simulink library "lib_rfsoc_fec"  (R2020b)
settings: Solver=VariableStepAuto  StartTime=0.0  StopTime=10.0  RelTol=1e-3
undefined symbols (not defined in the file): d, fs, generator_polynomial
libraries: hdlsllib x114, commseqgen3 x84, simulink x22, dspsigops x13, $bdroot x2
(part 4 of 5)

== system lib_rfsoc_fec/QAM Mapping/QAM Mapping/N-Width QAM-16 Symbol Mapping Imag/QAM-16 Symbol Mapping 11 ==
  bits : Inport
  Bit Slice1 : hdlsllib/Logic and Bit Operations/Bit Slice  lidx=n+1  ridx=n
      settings: SourceProductBaseCode=SL
  Constant1 : Constant  Value=3  OutDataTypeStr=fixdt(1,3,0)  SampleTime=-1
  Constant2 : Constant  OutDataTypeStr=fixdt(1,3,0)  SampleTime=-1
  Constant3 : Constant  Value=-1  OutDataTypeStr=fixdt(1,3,0)  SampleTime=-1
  Constant4 : Constant  Value=-3  OutDataTypeStr=fixdt(1,3,0)  SampleTime=-1
  Multiport Switch1 : MultiPortSwitch  DataPortOrder=Zero-based contiguous  Inputs=4  zeroidx=on
  Q : Outport
  wires:
  Bit Slice1/1 -> Multiport Switch1/1
  Multiport Switch1/1 -> Q/1
  bits/1 -> Bit Slice1/1
  Constant3/1 -> Multiport Switch1/5
  Constant4/1 -> Multiport Switch1/4
  Constant1/1 -> Multiport Switch1/2
  Constant2/1 -> Multiport Switch1/3

== system lib_rfsoc_fec/QAM Mapping/QAM Mapping/N-Width QAM-16 Symbol Mapping Imag/QAM-16 Symbol Mapping 12 ==
  bits : Inport
  Bit Slice1 : hdlsllib/Logic and Bit Operations/Bit Slice  lidx=n+1  ridx=n
      settings: SourceProductBaseCode=SL
  Constant1 : Constant  Value=3  OutDataTypeStr=fixdt(1,3,0)  SampleTime=-1
  Constant2 : Constant  OutDataTypeStr=fixdt(1,3,0)  SampleTime=-1
  Constant3 : Constant  Value=-1  OutDataTypeStr=fixdt(1,3,0)  SampleTime=-1
  Constant4 : Constant  Value=-3  OutDataTypeStr=fixdt(1,3,0)  SampleTime=-1
  Multiport Switch1 : MultiPortSwitch  DataPortOrder=Zero-based contiguous  Inputs=4  zeroidx=on
  Q : Outport
  wires:
  Bit Slice1/1 -> Multiport Switch1/1
  Multiport Switch1/1 -> Q/1
  bits/1 -> Bit Slice1/1
  Constant3/1 -> Multiport Switch1/5
  Constant4/1 -> Multiport Switch1/4
  Constant1/1 -> Multiport Switch1/2
  Constant2/1 -> Multiport Switch1/3

== system lib_rfsoc_fec/QAM Mapping/QAM Mapping/N-Width QAM-16 Symbol Mapping Imag/QAM-16 Symbol Mapping 13 ==
  bits : Inport
  Bit Slice1 : hdlsllib/Logic and Bit Operations/Bit Slice  lidx=n+1  ridx=n
      settings: SourceProductBaseCode=SL
  Constant1 : Constant  Value=3  OutDataTypeStr=fixdt(1,3,0)  SampleTime=-1
  Constant2 : Constant  OutDataTypeStr=fixdt(1,3,0)  SampleTime=-1
  Constant3 : Constant  Value=-1  OutDataTypeStr=fixdt(1,3,0)  SampleTime=-1
  Constant4 : Constant  Value=-3  OutDataTypeStr=fixdt(1,3,0)  SampleTime=-1
  Multiport Switch1 : MultiPortSwitch  DataPortOrder=Zero-based contiguous  Inputs=4  zeroidx=on
  Q : Outport
  wires:
  Bit Slice1/1 -> Multiport Switch1/1
  Multiport Switch1/1 -> Q/1
  bits/1 -> Bit Slice1/1
  Constant3/1 -> Multiport Switch1/5
  Constant4/1 -> Multiport Switch1/4
  Constant1/1 -> Multiport Switch1/2
  Constant2/1 -> Multiport Switch1/3

== system lib_rfsoc_fec/QAM Mapping/QAM Mapping/N-Width QAM-16 Symbol Mapping Imag/QAM-16 Symbol Mapping 14 ==
  bits : Inport
  Bit Slice1 : hdlsllib/Logic and Bit Operations/Bit Slice  lidx=n+1  ridx=n
      settings: SourceProductBaseCode=SL
  Constant1 : Constant  Value=3  OutDataTypeStr=fixdt(1,3,0)  SampleTime=-1
  Constant2 : Constant  OutDataTypeStr=fixdt(1,3,0)  SampleTime=-1
  Constant3 : Constant  Value=-1  OutDataTypeStr=fixdt(1,3,0)  SampleTime=-1
  Constant4 : Constant  Value=-3  OutDataTypeStr=fixdt(1,3,0)  SampleTime=-1
  Multiport Switch1 : MultiPortSwitch  DataPortOrder=Zero-based contiguous  Inputs=4  zeroidx=on
  Q : Outport
  wires:
  Bit Slice1/1 -> Multiport Switch1/1
  Multiport Switch1/1 -> Q/1
  bits/1 -> Bit Slice1/1
  Constant3/1 -> Multiport Switch1/5
  Constant4/1 -> Multiport Switch1/4
  Constant1/1 -> Multiport Switch1/2
  Constant2/1 -> Multiport Switch1/3

== system lib_rfsoc_fec/QAM Mapping/QAM Mapping/N-Width QAM-16 Symbol Mapping Imag/QAM-16 Symbol Mapping 15 ==
  bits : Inport
  Bit Slice1 : hdlsllib/Logic and Bit Operations/Bit Slice  lidx=n+1  ridx=n
      settings: SourceProductBaseCode=SL
  Constant1 : Constant  Value=3  OutDataTypeStr=fixdt(1,3,0)  SampleTime=-1
  Constant2 : Constant  OutDataTypeStr=fixdt(1,3,0)  SampleTime=-1
  Constant3 : Constant  Value=-1  OutDataTypeStr=fixdt(1,3,0)  SampleTime=-1
  Constant4 : Constant  Value=-3  OutDataTypeStr=fixdt(1,3,0)  SampleTime=-1
  Multiport Switch1 : MultiPortSwitch  DataPortOrder=Zero-based contiguous  Inputs=4  zeroidx=on
  Q : Outport
  wires:
  Bit Slice1/1 -> Multiport Switch1/1
  Multiport Switch1/1 -> Q/1
  bits/1 -> Bit Slice1/1
  Constant3/1 -> Multiport Switch1/5
  Constant4/1 -> Multiport Switch1/4
  Constant1/1 -> Multiport Switch1/2
  Constant2/1 -> Multiport Switch1/3

== system lib_rfsoc_fec/QAM Mapping/QAM Mapping/N-Width QAM-16 Symbol Mapping Imag/QAM-16 Symbol Mapping 16 ==
  bits : Inport
  Bit Slice1 : hdlsllib/Logic and Bit Operations/Bit Slice  lidx=n+1  ridx=n
      settings: SourceProductBaseCode=SL
  Constant1 : Constant  Value=3  OutDataTypeStr=fixdt(1,3,0)  SampleTime=-1
  Constant2 : Constant  OutDataTypeStr=fixdt(1,3,0)  SampleTime=-1
  Constant3 : Constant  Value=-1  OutDataTypeStr=fixdt(1,3,0)  SampleTime=-1
  Constant4 : Constant  Value=-3  OutDataTypeStr=fixdt(1,3,0)  SampleTime=-1
  Multiport Switch1 : MultiPortSwitch  DataPortOrder=Zero-based contiguous  Inputs=4  zeroidx=on
  Q : Outport
  wires:
  Bit Slice1/1 -> Multiport Switch1/1
  Multiport Switch1/1 -> Q/1
  bits/1 -> Bit Slice1/1
  Constant3/1 -> Multiport Switch1/5
  Constant4/1 -> Multiport Switch1/4
  Constant1/1 -> Multiport Switch1/2
  Constant2/1 -> Multiport Switch1/3

== system lib_rfsoc_fec/QAM Mapping/QAM Mapping/N-Width QAM-16 Symbol Mapping Imag/QAM-16 Symbol Mapping 17 ==
  bits : Inport
  Bit Slice1 : hdlsllib/Logic and Bit Operations/Bit Slice  lidx=n+1  ridx=n
      settings: SourceProductBaseCode=SL
  Constant1 : Constant  Value=3  OutDataTypeStr=fixdt(1,3,0)  SampleTime=-1
  Constant2 : Constant  OutDataTypeStr=fixdt(1,3,0)  SampleTime=-1
  Constant3 : Constant  Value=-1  OutDataTypeStr=fixdt(1,3,0)  SampleTime=-1
  Constant4 : Constant  Value=-3  OutDataTypeStr=fixdt(1,3,0)  SampleTime=-1
  Multiport Switch1 : MultiPortSwitch  DataPortOrder=Zero-based contiguous  Inputs=4  zeroidx=on
  Q : Outport
  wires:
  Bit Slice1/1 -> Multiport Switch1/1
  Multiport Switch1/1 -> Q/1
  bits/1 -> Bit Slice1/1
  Constant3/1 -> Multiport Switch1/5
  Constant4/1 -> Multiport Switch1/4
  Constant1/1 -> Multiport Switch1/2
  Constant2/1 -> Multiport Switch1/3

== system lib_rfsoc_fec/QAM Mapping/QAM Mapping/N-Width QAM-16 Symbol Mapping Imag/QAM-16 Symbol Mapping 18 ==
  bits : Inport
  Bit Slice1 : hdlsllib/Logic and Bit Operations/Bit Slice  lidx=n+1  ridx=n
      settings: SourceProductBaseCode=SL
  Constant1 : Constant  Value=3  OutDataTypeStr=fixdt(1,3,0)  SampleTime=-1
  Constant2 : Constant  OutDataTypeStr=fixdt(1,3,0)  SampleTime=-1
  Constant3 : Constant  Value=-1  OutDataTypeStr=fixdt(1,3,0)  SampleTime=-1
  Constant4 : Constant  Value=-3  OutDataTypeStr=fixdt(1,3,0)  SampleTime=-1
  Multiport Switch1 : MultiPortSwitch  DataPortOrder=Zero-based contiguous  Inputs=4  zeroidx=on
  Q : Outport
  wires:
  Bit Slice1/1 -> Multiport Switch1/1
  Multiport Switch1/1 -> Q/1
  bits/1 -> Bit Slice1/1
  Constant3/1 -> Multiport Switch1/5
  Constant4/1 -> Multiport Switch1/4
  Constant1/1 -> Multiport Switch1/2
  Constant2/1 -> Multiport Switch1/3

== system lib_rfsoc_fec/QAM Mapping/QAM Mapping/N-Width QAM-16 Symbol Mapping Imag/QAM-16 Symbol Mapping 19 ==
  bits : Inport
  Bit Slice1 : hdlsllib/Logic and Bit Operations/Bit Slice  lidx=n+1  ridx=n
      settings: SourceProductBaseCode=SL
  Constant1 : Constant  Value=3  OutDataTypeStr=fixdt(1,3,0)  SampleTime=-1
  Constant2 : Constant  OutDataTypeStr=fixdt(1,3,0)  SampleTime=-1
  Constant3 : Constant  Value=-1  OutDataTypeStr=fixdt(1,3,0)  SampleTime=-1
  Constant4 : Constant  Value=-3  OutDataTypeStr=fixdt(1,3,0)  SampleTime=-1
  Multiport Switch1 : MultiPortSwitch  DataPortOrder=Zero-based contiguous  Inputs=4  zeroidx=on
  Q : Outport
  wires:
  Bit Slice1/1 -> Multiport Switch1/1
  Multiport Switch1/1 -> Q/1
  bits/1 -> Bit Slice1/1
  Constant3/1 -> Multiport Switch1/5
  Constant4/1 -> Multiport Switch1/4
  Constant1/1 -> Multiport Switch1/2
  Constant2/1 -> Multiport Switch1/3

== system lib_rfsoc_fec/QAM Mapping/QAM Mapping/N-Width QAM-16 Symbol Mapping Imag/QAM-16 Symbol Mapping 2 ==
  bits : Inport
  Bit Slice1 : hdlsllib/Logic and Bit Operations/Bit Slice  lidx=n+1  ridx=n
      settings: SourceProductBaseCode=SL
  Constant1 : Constant  Value=3  OutDataTypeStr=fixdt(1,3,0)  SampleTime=-1
  Constant2 : Constant  OutDataTypeStr=fixdt(1,3,0)  SampleTime=-1
  Constant3 : Constant  Value=-1  OutDataTypeStr=fixdt(1,3,0)  SampleTime=-1
  Constant4 : Constant  Value=-3  OutDataTypeStr=fixdt(1,3,0)  SampleTime=-1
  Multiport Switch1 : MultiPortSwitch  DataPortOrder=Zero-based contiguous  Inputs=4  zeroidx=on
  Q : Outport
  wires:
  Bit Slice1/1 -> Multiport Switch1/1
  Multiport Switch1/1 -> Q/1
  bits/1 -> Bit Slice1/1
  Constant3/1 -> Multiport Switch1/5
  Constant4/1 -> Multiport Switch1/4
  Constant1/1 -> Multiport Switch1/2
  Constant2/1 -> Multiport Switch1/3

== system lib_rfsoc_fec/QAM Mapping/QAM Mapping/N-Width QAM-16 Symbol Mapping Imag/QAM-16 Symbol Mapping 20 ==
  bits : Inport
  Bit Slice1 : hdlsllib/Logic and Bit Operations/Bit Slice  lidx=n+1  ridx=n
      settings: SourceProductBaseCode=SL
  Constant1 : Constant  Value=3  OutDataTypeStr=fixdt(1,3,0)  SampleTime=-1
  Constant2 : Constant  OutDataTypeStr=fixdt(1,3,0)  SampleTime=-1
  Constant3 : Constant  Value=-1  OutDataTypeStr=fixdt(1,3,0)  SampleTime=-1
  Constant4 : Constant  Value=-3  OutDataTypeStr=fixdt(1,3,0)  SampleTime=-1
  Multiport Switch1 : MultiPortSwitch  DataPortOrder=Zero-based contiguous  Inputs=4  zeroidx=on
  Q : Outport
  wires:
  Bit Slice1/1 -> Multiport Switch1/1
  Multiport Switch1/1 -> Q/1
  bits/1 -> Bit Slice1/1
  Constant3/1 -> Multiport Switch1/5
  Constant4/1 -> Multiport Switch1/4
  Constant1/1 -> Multiport Switch1/2
  Constant2/1 -> Multiport Switch1/3

== system lib_rfsoc_fec/QAM Mapping/QAM Mapping/N-Width QAM-16 Symbol Mapping Imag/QAM-16 Symbol Mapping 21 ==
  bits : Inport
  Bit Slice1 : hdlsllib/Logic and Bit Operations/Bit Slice  lidx=n+1  ridx=n
      settings: SourceProductBaseCode=SL
  Constant1 : Constant  Value=3  OutDataTypeStr=fixdt(1,3,0)  SampleTime=-1
  Constant2 : Constant  OutDataTypeStr=fixdt(1,3,0)  SampleTime=-1
  Constant3 : Constant  Value=-1  OutDataTypeStr=fixdt(1,3,0)  SampleTime=-1
  Constant4 : Constant  Value=-3  OutDataTypeStr=fixdt(1,3,0)  SampleTime=-1
  Multiport Switch1 : MultiPortSwitch  DataPortOrder=Zero-based contiguous  Inputs=4  zeroidx=on
  Q : Outport
  wires:
  Bit Slice1/1 -> Multiport Switch1/1
  Multiport Switch1/1 -> Q/1
  bits/1 -> Bit Slice1/1
  Constant3/1 -> Multiport Switch1/5
  Constant4/1 -> Multiport Switch1/4
  Constant1/1 -> Multiport Switch1/2
  Constant2/1 -> Multiport Switch1/3

== system lib_rfsoc_fec/QAM Mapping/QAM Mapping/N-Width QAM-16 Symbol Mapping Imag/QAM-16 Symbol Mapping 22 ==
  bits : Inport
  Bit Slice1 : hdlsllib/Logic and Bit Operations/Bit Slice  lidx=n+1  ridx=n
      settings: SourceProductBaseCode=SL
  Constant1 : Constant  Value=3  OutDataTypeStr=fixdt(1,3,0)  SampleTime=-1
  Constant2 : Constant  OutDataTypeStr=fixdt(1,3,0)  SampleTime=-1
  Constant3 : Constant  Value=-1  OutDataTypeStr=fixdt(1,3,0)  SampleTime=-1
  Constant4 : Constant  Value=-3  OutDataTypeStr=fixdt(1,3,0)  SampleTime=-1
  Multiport Switch1 : MultiPortSwitch  DataPortOrder=Zero-based contiguous  Inputs=4  zeroidx=on
  Q : Outport
  wires:
  Bit Slice1/1 -> Multiport Switch1/1
  Multiport Switch1/1 -> Q/1
  bits/1 -> Bit Slice1/1
  Constant3/1 -> Multiport Switch1/5
  Constant4/1 -> Multiport Switch1/4
  Constant1/1 -> Multiport Switch1/2
  Constant2/1 -> Multiport Switch1/3

== system lib_rfsoc_fec/QAM Mapping/QAM Mapping/N-Width QAM-16 Symbol Mapping Imag/QAM-16 Symbol Mapping 23 ==
  bits : Inport
  Bit Slice1 : hdlsllib/Logic and Bit Operations/Bit Slice  lidx=n+1  ridx=n
      settings: SourceProductBaseCode=SL
  Constant1 : Constant  Value=3  OutDataTypeStr=fixdt(1,3,0)  SampleTime=-1
  Constant2 : Constant  OutDataTypeStr=fixdt(1,3,0)  SampleTime=-1
  Constant3 : Constant  Value=-1  OutDataTypeStr=fixdt(1,3,0)  SampleTime=-1
  Constant4 : Constant  Value=-3  OutDataTypeStr=fixdt(1,3,0)  SampleTime=-1
  Multiport Switch1 : MultiPortSwitch  DataPortOrder=Zero-based contiguous  Inputs=4  zeroidx=on
  Q : Outport
  wires:
  Bit Slice1/1 -> Multiport Switch1/1
  Multiport Switch1/1 -> Q/1
  bits/1 -> Bit Slice1/1
  Constant3/1 -> Multiport Switch1/5
  Constant4/1 -> Multiport Switch1/4
  Constant1/1 -> Multiport Switch1/2
  Constant2/1 -> Multiport Switch1/3

== system lib_rfsoc_fec/QAM Mapping/QAM Mapping/N-Width QAM-16 Symbol Mapping Imag/QAM-16 Symbol Mapping 24 ==
  bits : Inport
  Bit Slice1 : hdlsllib/Logic and Bit Operations/Bit Slice  lidx=n+1  ridx=n
      settings: SourceProductBaseCode=SL
  Constant1 : Constant  Value=3  OutDataTypeStr=fixdt(1,3,0)  SampleTime=-1
  Constant2 : Constant  OutDataTypeStr=fixdt(1,3,0)  SampleTime=-1
  Constant3 : Constant  Value=-1  OutDataTypeStr=fixdt(1,3,0)  SampleTime=-1
  Constant4 : Constant  Value=-3  OutDataTypeStr=fixdt(1,3,0)  SampleTime=-1
  Multiport Switch1 : MultiPortSwitch  DataPortOrder=Zero-based contiguous  Inputs=4  zeroidx=on
  Q : Outport
  wires:
  Bit Slice1/1 -> Multiport Switch1/1
  Multiport Switch1/1 -> Q/1
  bits/1 -> Bit Slice1/1
  Constant3/1 -> Multiport Switch1/5
  Constant4/1 -> Multiport Switch1/4
  Constant1/1 -> Multiport Switch1/2
  Constant2/1 -> Multiport Switch1/3

== system lib_rfsoc_fec/QAM Mapping/QAM Mapping/N-Width QAM-16 Symbol Mapping Imag/QAM-16 Symbol Mapping 25 ==
  bits : Inport
  Bit Slice1 : hdlsllib/Logic and Bit Operations/Bit Slice  lidx=n+1  ridx=n
      settings: SourceProductBaseCode=SL
  Constant1 : Constant  Value=3  OutDataTypeStr=fixdt(1,3,0)  SampleTime=-1
  Constant2 : Constant  OutDataTypeStr=fixdt(1,3,0)  SampleTime=-1
  Constant3 : Constant  Value=-1  OutDataTypeStr=fixdt(1,3,0)  SampleTime=-1
  Constant4 : Constant  Value=-3  OutDataTypeStr=fixdt(1,3,0)  SampleTime=-1
  Multiport Switch1 : MultiPortSwitch  DataPortOrder=Zero-based contiguous  Inputs=4  zeroidx=on
  Q : Outport
  wires:
  Bit Slice1/1 -> Multiport Switch1/1
  Multiport Switch1/1 -> Q/1
  bits/1 -> Bit Slice1/1
  Constant3/1 -> Multiport Switch1/5
  Constant4/1 -> Multiport Switch1/4
  Constant1/1 -> Multiport Switch1/2
  Constant2/1 -> Multiport Switch1/3

== system lib_rfsoc_fec/QAM Mapping/QAM Mapping/N-Width QAM-16 Symbol Mapping Imag/QAM-16 Symbol Mapping 26 ==
  bits : Inport
  Bit Slice1 : hdlsllib/Logic and Bit Operations/Bit Slice  lidx=n+1  ridx=n
      settings: SourceProductBaseCode=SL
  Constant1 : Constant  Value=3  OutDataTypeStr=fixdt(1,3,0)  SampleTime=-1
  Constant2 : Constant  OutDataTypeStr=fixdt(1,3,0)  SampleTime=-1
  Constant3 : Constant  Value=-1  OutDataTypeStr=fixdt(1,3,0)  SampleTime=-1
  Constant4 : Constant  Value=-3  OutDataTypeStr=fixdt(1,3,0)  SampleTime=-1
  Multiport Switch1 : MultiPortSwitch  DataPortOrder=Zero-based contiguous  Inputs=4  zeroidx=on
  Q : Outport
  wires:
  Bit Slice1/1 -> Multiport Switch1/1
  Multiport Switch1/1 -> Q/1
  bits/1 -> Bit Slice1/1
  Constant3/1 -> Multiport Switch1/5
  Constant4/1 -> Multiport Switch1/4
  Constant1/1 -> Multiport Switch1/2
  Constant2/1 -> Multiport Switch1/3

== system lib_rfsoc_fec/QAM Mapping/QAM Mapping/N-Width QAM-16 Symbol Mapping Imag/QAM-16 Symbol Mapping 27 ==
  bits : Inport
  Bit Slice1 : hdlsllib/Logic and Bit Operations/Bit Slice  lidx=n+1  ridx=n
      settings: SourceProductBaseCode=SL
  Constant1 : Constant  Value=3  OutDataTypeStr=fixdt(1,3,0)  SampleTime=-1
  Constant2 : Constant  OutDataTypeStr=fixdt(1,3,0)  SampleTime=-1
  Constant3 : Constant  Value=-1  OutDataTypeStr=fixdt(1,3,0)  SampleTime=-1
  Constant4 : Constant  Value=-3  OutDataTypeStr=fixdt(1,3,0)  SampleTime=-1
  Multiport Switch1 : MultiPortSwitch  DataPortOrder=Zero-based contiguous  Inputs=4  zeroidx=on
  Q : Outport
  wires:
  Bit Slice1/1 -> Multiport Switch1/1
  Multiport Switch1/1 -> Q/1
  bits/1 -> Bit Slice1/1
  Constant3/1 -> Multiport Switch1/5
  Constant4/1 -> Multiport Switch1/4
  Constant1/1 -> Multiport Switch1/2
  Constant2/1 -> Multiport Switch1/3

== system lib_rfsoc_fec/QAM Mapping/QAM Mapping/N-Width QAM-16 Symbol Mapping Imag/QAM-16 Symbol Mapping 28 ==
  bits : Inport
  Bit Slice1 : hdlsllib/Logic and Bit Operations/Bit Slice  lidx=n+1  ridx=n
      settings: SourceProductBaseCode=SL
  Constant1 : Constant  Value=3  OutDataTypeStr=fixdt(1,3,0)  SampleTime=-1
  Constant2 : Constant  OutDataTypeStr=fixdt(1,3,0)  SampleTime=-1
  Constant3 : Constant  Value=-1  OutDataTypeStr=fixdt(1,3,0)  SampleTime=-1
  Constant4 : Constant  Value=-3  OutDataTypeStr=fixdt(1,3,0)  SampleTime=-1
  Multiport Switch1 : MultiPortSwitch  DataPortOrder=Zero-based contiguous  Inputs=4  zeroidx=on
  Q : Outport
  wires:
  Bit Slice1/1 -> Multiport Switch1/1
  Multiport Switch1/1 -> Q/1
  bits/1 -> Bit Slice1/1
  Constant3/1 -> Multiport Switch1/5
  Constant4/1 -> Multiport Switch1/4
  Constant1/1 -> Multiport Switch1/2
  Constant2/1 -> Multiport Switch1/3

== system lib_rfsoc_fec/QAM Mapping/QAM Mapping/N-Width QAM-16 Symbol Mapping Imag/QAM-16 Symbol Mapping 29 ==
  bits : Inport
  Bit Slice1 : hdlsllib/Logic and Bit Operations/Bit Slice  lidx=n+1  ridx=n
      settings: SourceProductBaseCode=SL
  Constant1 : Constant  Value=3  OutDataTypeStr=fixdt(1,3,0)  SampleTime=-1
  Constant2 : Constant  OutDataTypeStr=fixdt(1,3,0)  SampleTime=-1
  Constant3 : Constant  Value=-1  OutDataTypeStr=fixdt(1,3,0)  SampleTime=-1
  Constant4 : Constant  Value=-3  OutDataTypeStr=fixdt(1,3,0)  SampleTime=-1
  Multiport Switch1 : MultiPortSwitch  DataPortOrder=Zero-based contiguous  Inputs=4  zeroidx=on
  Q : Outport
  wires:
  Bit Slice1/1 -> Multiport Switch1/1
  Multiport Switch1/1 -> Q/1
  bits/1 -> Bit Slice1/1
  Constant3/1 -> Multiport Switch1/5
  Constant4/1 -> Multiport Switch1/4
  Constant1/1 -> Multiport Switch1/2
  Constant2/1 -> Multiport Switch1/3

== system lib_rfsoc_fec/QAM Mapping/QAM Mapping/N-Width QAM-16 Symbol Mapping Imag/QAM-16 Symbol Mapping 3 ==
  bits : Inport
  Bit Slice1 : hdlsllib/Logic and Bit Operations/Bit Slice  lidx=n+1  ridx=n
      settings: SourceProductBaseCode=SL
  Constant1 : Constant  Value=3  OutDataTypeStr=fixdt(1,3,0)  SampleTime=-1
  Constant2 : Constant  OutDataTypeStr=fixdt(1,3,0)  SampleTime=-1
  Constant3 : Constant  Value=-1  OutDataTypeStr=fixdt(1,3,0)  SampleTime=-1
  Constant4 : Constant  Value=-3  OutDataTypeStr=fixdt(1,3,0)  SampleTime=-1
  Multiport Switch1 : MultiPortSwitch  DataPortOrder=Zero-based contiguous  Inputs=4  zeroidx=on
  Q : Outport
  wires:
  Bit Slice1/1 -> Multiport Switch1/1
  Multiport Switch1/1 -> Q/1
  bits/1 -> Bit Slice1/1
  Constant3/1 -> Multiport Switch1/5
  Constant4/1 -> Multiport Switch1/4
  Constant1/1 -> Multiport Switch1/2
  Constant2/1 -> Multiport Switch1/3

== system lib_rfsoc_fec/QAM Mapping/QAM Mapping/N-Width QAM-16 Symbol Mapping Imag/QAM-16 Symbol Mapping 30 ==
  bits : Inport
  Bit Slice1 : hdlsllib/Logic and Bit Operations/Bit Slice  lidx=n+1  ridx=n
      settings: SourceProductBaseCode=SL
  Constant1 : Constant  Value=3  OutDataTypeStr=fixdt(1,3,0)  SampleTime=-1
  Constant2 : Constant  OutDataTypeStr=fixdt(1,3,0)  SampleTime=-1
  Constant3 : Constant  Value=-1  OutDataTypeStr=fixdt(1,3,0)  SampleTime=-1
  Constant4 : Constant  Value=-3  OutDataTypeStr=fixdt(1,3,0)  SampleTime=-1
  Multiport Switch1 : MultiPortSwitch  DataPortOrder=Zero-based contiguous  Inputs=4  zeroidx=on
  Q : Outport
  wires:
  Bit Slice1/1 -> Multiport Switch1/1
  Multiport Switch1/1 -> Q/1
  bits/1 -> Bit Slice1/1
  Constant3/1 -> Multiport Switch1/5
  Constant4/1 -> Multiport Switch1/4
  Constant1/1 -> Multiport Switch1/2
  Constant2/1 -> Multiport Switch1/3

== system lib_rfsoc_fec/QAM Mapping/QAM Mapping/N-Width QAM-16 Symbol Mapping Imag/QAM-16 Symbol Mapping 31 ==
  bits : Inport
  Bit Slice1 : hdlsllib/Logic and Bit Operations/Bit Slice  lidx=n+1  ridx=n
      settings: SourceProductBaseCode=SL
  Constant1 : Constant  Value=3  OutDataTypeStr=fixdt(1,3,0)  SampleTime=-1
  Constant2 : Constant  OutDataTypeStr=fixdt(1,3,0)  SampleTime=-1
  Constant3 : Constant  Value=-1  OutDataTypeStr=fixdt(1,3,0)  SampleTime=-1
  Constant4 : Constant  Value=-3  OutDataTypeStr=fixdt(1,3,0)  SampleTime=-1
  Multiport Switch1 : MultiPortSwitch  DataPortOrder=Zero-based contiguous  Inputs=4  zeroidx=on
  Q : Outport
  wires:
  Bit Slice1/1 -> Multiport Switch1/1
  Multiport Switch1/1 -> Q/1
  bits/1 -> Bit Slice1/1
  Constant3/1 -> Multiport Switch1/5
  Constant4/1 -> Multiport Switch1/4
  Constant1/1 -> Multiport Switch1/2
  Constant2/1 -> Multiport Switch1/3

== system lib_rfsoc_fec/QAM Mapping/QAM Mapping/N-Width QAM-16 Symbol Mapping Imag/QAM-16 Symbol Mapping 4 ==
  bits : Inport
  Bit Slice1 : hdlsllib/Logic and Bit Operations/Bit Slice  lidx=n+1  ridx=n
      settings: SourceProductBaseCode=SL
  Constant1 : Constant  Value=3  OutDataTypeStr=fixdt(1,3,0)  SampleTime=-1
  Constant2 : Constant  OutDataTypeStr=fixdt(1,3,0)  SampleTime=-1
  Constant3 : Constant  Value=-1  OutDataTypeStr=fixdt(1,3,0)  SampleTime=-1
  Constant4 : Constant  Value=-3  OutDataTypeStr=fixdt(1,3,0)  SampleTime=-1
  Multiport Switch1 : MultiPortSwitch  DataPortOrder=Zero-based contiguous  Inputs=4  zeroidx=on
  Q : Outport
  wires:
  Bit Slice1/1 -> Multiport Switch1/1
  Multiport Switch1/1 -> Q/1
  bits/1 -> Bit Slice1/1
  Constant3/1 -> Multiport Switch1/5
  Constant4/1 -> Multiport Switch1/4
  Constant1/1 -> Multiport Switch1/2
  Constant2/1 -> Multiport Switch1/3

== system lib_rfsoc_fec/QAM Mapping/QAM Mapping/N-Width QAM-16 Symbol Mapping Imag/QAM-16 Symbol Mapping 5 ==
  bits : Inport
  Bit Slice1 : hdlsllib/Logic and Bit Operations/Bit Slice  lidx=n+1  ridx=n
      settings: SourceProductBaseCode=SL
  Constant1 : Constant  Value=3  OutDataTypeStr=fixdt(1,3,0)  SampleTime=-1
  Constant2 : Constant  OutDataTypeStr=fixdt(1,3,0)  SampleTime=-1
  Constant3 : Constant  Value=-1  OutDataTypeStr=fixdt(1,3,0)  SampleTime=-1
  Constant4 : Constant  Value=-3  OutDataTypeStr=fixdt(1,3,0)  SampleTime=-1
  Multiport Switch1 : MultiPortSwitch  DataPortOrder=Zero-based contiguous  Inputs=4  zeroidx=on
  Q : Outport
  wires:
  Bit Slice1/1 -> Multiport Switch1/1
  Multiport Switch1/1 -> Q/1
  bits/1 -> Bit Slice1/1
  Constant3/1 -> Multiport Switch1/5
  Constant4/1 -> Multiport Switch1/4
  Constant1/1 -> Multiport Switch1/2
  Constant2/1 -> Multiport Switch1/3

== system lib_rfsoc_fec/QAM Mapping/QAM Mapping/N-Width QAM-16 Symbol Mapping Imag/QAM-16 Symbol Mapping 6 ==
  bits : Inport
  Bit Slice1 : hdlsllib/Logic and Bit Operations/Bit Slice  lidx=n+1  ridx=n
      settings: SourceProductBaseCode=SL
  Constant1 : Constant  Value=3  OutDataTypeStr=fixdt(1,3,0)  SampleTime=-1
  Constant2 : Constant  OutDataTypeStr=fixdt(1,3,0)  SampleTime=-1
  Constant3 : Constant  Value=-1  OutDataTypeStr=fixdt(1,3,0)  SampleTime=-1
  Constant4 : Constant  Value=-3  OutDataTypeStr=fixdt(1,3,0)  SampleTime=-1
  Multiport Switch1 : MultiPortSwitch  DataPortOrder=Zero-based contiguous  Inputs=4  zeroidx=on
  Q : Outport
  wires:
  Bit Slice1/1 -> Multiport Switch1/1
  Multiport Switch1/1 -> Q/1
  bits/1 -> Bit Slice1/1
  Constant3/1 -> Multiport Switch1/5
  Constant4/1 -> Multiport Switch1/4
  Constant1/1 -> Multiport Switch1/2
  Constant2/1 -> Multiport Switch1/3

== system lib_rfsoc_fec/QAM Mapping/QAM Mapping/N-Width QAM-16 Symbol Mapping Imag/QAM-16 Symbol Mapping 7 ==
  bits : Inport
  Bit Slice1 : hdlsllib/Logic and Bit Operations/Bit Slice  lidx=n+1  ridx=n
      settings: SourceProductBaseCode=SL
  Constant1 : Constant  Value=3  OutDataTypeStr=fixdt(1,3,0)  SampleTime=-1
  Constant2 : Constant  OutDataTypeStr=fixdt(1,3,0)  SampleTime=-1
  Constant3 : Constant  Value=-1  OutDataTypeStr=fixdt(1,3,0)  SampleTime=-1
  Constant4 : Constant  Value=-3  OutDataTypeStr=fixdt(1,3,0)  SampleTime=-1
  Multiport Switch1 : MultiPortSwitch  DataPortOrder=Zero-based contiguous  Inputs=4  zeroidx=on
  Q : Outport
  wires:
  Bit Slice1/1 -> Multiport Switch1/1
  Multiport Switch1/1 -> Q/1
  bits/1 -> Bit Slice1/1
  Constant3/1 -> Multiport Switch1/5
  Constant4/1 -> Multiport Switch1/4
  Constant1/1 -> Multiport Switch1/2
  Constant2/1 -> Multiport Switch1/3

== system lib_rfsoc_fec/QAM Mapping/QAM Mapping/N-Width QAM-16 Symbol Mapping Imag/QAM-16 Symbol Mapping 8 ==
  bits : Inport
  Bit Slice1 : hdlsllib/Logic and Bit Operations/Bit Slice  lidx=n+1  ridx=n
      settings: SourceProductBaseCode=SL
  Constant1 : Constant  Value=3  OutDataTypeStr=fixdt(1,3,0)  SampleTime=-1
  Constant2 : Constant  OutDataTypeStr=fixdt(1,3,0)  SampleTime=-1
  Constant3 : Constant  Value=-1  OutDataTypeStr=fixdt(1,3,0)  SampleTime=-1
  Constant4 : Constant  Value=-3  OutDataTypeStr=fixdt(1,3,0)  SampleTime=-1
  Multiport Switch1 : MultiPortSwitch  DataPortOrder=Zero-based contiguous  Inputs=4  zeroidx=on
  Q : Outport
  wires:
  Bit Slice1/1 -> Multiport Switch1/1
  Multiport Switch1/1 -> Q/1
  bits/1 -> Bit Slice1/1
  Constant3/1 -> Multiport Switch1/5
  Constant4/1 -> Multiport Switch1/4
  Constant1/1 -> Multiport Switch1/2
  Constant2/1 -> Multiport Switch1/3

== system lib_rfsoc_fec/QAM Mapping/QAM Mapping/N-Width QAM-16 Symbol Mapping Imag/QAM-16 Symbol Mapping 9 ==
  bits : Inport
  Bit Slice1 : hdlsllib/Logic and Bit Operations/Bit Slice  lidx=n+1  ridx=n
      settings: SourceProductBaseCode=SL
  Constant1 : Constant  Value=3  OutDataTypeStr=fixdt(1,3,0)  SampleTime=-1
  Constant2 : Constant  OutDataTypeStr=fixdt(1,3,0)  SampleTime=-1
  Constant3 : Constant  Value=-1  OutDataTypeStr=fixdt(1,3,0)  SampleTime=-1
  Constant4 : Constant  Value=-3  OutDataTypeStr=fixdt(1,3,0)  SampleTime=-1
  Multiport Switch1 : MultiPortSwitch  DataPortOrder=Zero-based contiguous  Inputs=4  zeroidx=on
  Q : Outport
  wires:
  Bit Slice1/1 -> Multiport Switch1/1
  Multiport Switch1/1 -> Q/1
  bits/1 -> Bit Slice1/1
  Constant3/1 -> Multiport Switch1/5
  Constant4/1 -> Multiport Switch1/4
  Constant1/1 -> Multiport Switch1/2
  Constant2/1 -> Multiport Switch1/3

== system lib_rfsoc_fec/QAM Mapping/QAM Mapping/N-Width QAM-16 Symbol Mapping Real/QAM-16 Symbol Mapping 0 ==
  bits : Inport
  Bit Slice2 : hdlsllib/Logic and Bit Operations/Bit Slice  lidx=n+3  ridx=n+2
      settings: SourceProductBaseCode=SL
  Constant1 : Constant  Value=3  OutDataTypeStr=fixdt(1,3,0)  SampleTime=-1
  Constant2 : Constant  OutDataTypeStr=fixdt(1,3,0)  SampleTime=-1
  Constant3 : Constant  Value=-1  OutDataTypeStr=fixdt(1,3,0)  SampleTime=-1
  Constant4 : Constant  Value=-3  OutDataTypeStr=fixdt(1,3,0)  SampleTime=-1
  Multiport Switch : MultiPortSwitch  DataPortOrder=Zero-based contiguous  Inputs=4  zeroidx=on
  I : Outport
  wires:
  Multiport Switch/1 -> I/1
  Constant2/1 -> Multiport Switch/5
  Constant1/1 -> Multiport Switch/4
  Constant4/1 -> Multiport Switch/2
  Constant3/1 -> Multiport Switch/3
  bits/1 -> Bit Slice2/1
  Bit Slice2/1 -> Multiport Switch/1

== system lib_rfsoc_fec/QAM Mapping/QAM Mapping/N-Width QAM-16 Symbol Mapping Real/QAM-16 Symbol Mapping 1 ==
  bits : Inport
  Bit Slice2 : hdlsllib/Logic and Bit Operations/Bit Slice  lidx=n+3  ridx=n+2
      settings: SourceProductBaseCode=SL
  Constant1 : Constant  Value=3  OutDataTypeStr=fixdt(1,3,0)  SampleTime=-1
  Constant2 : Constant  OutDataTypeStr=fixdt(1,3,0)  SampleTime=-1
  Constant3 : Constant  Value=-1  OutDataTypeStr=fixdt(1,3,0)  SampleTime=-1
  Constant4 : Constant  Value=-3  OutDataTypeStr=fixdt(1,3,0)  SampleTime=-1
  Multiport Switch : MultiPortSwitch  DataPortOrder=Zero-based contiguous  Inputs=4  zeroidx=on
  I : Outport
  wires:
  Bit Slice2/1 -> Multiport Switch/1
  bits/1 -> Bit Slice2/1
  Constant3/1 -> Multiport Switch/3
  Constant4/1 -> Multiport Switch/2
  Constant1/1 -> Multiport Switch/4
  Constant2/1 -> Multiport Switch/5
  Multiport Switch/1 -> I/1

== system lib_rfsoc_fec/QAM Mapping/QAM Mapping/N-Width QAM-16 Symbol Mapping Real/QAM-16 Symbol Mapping 10 ==
  bits : Inport
  Bit Slice2 : hdlsllib/Logic and Bit Operations/Bit Slice  lidx=n+3  ridx=n+2
      settings: SourceProductBaseCode=SL
  Constant1 : Constant  Value=3  OutDataTypeStr=fixdt(1,3,0)  SampleTime=-1
  Constant2 : Constant  OutDataTypeStr=fixdt(1,3,0)  SampleTime=-1
  Constant3 : Constant  Value=-1  OutDataTypeStr=fixdt(1,3,0)  SampleTime=-1
  Constant4 : Constant  Value=-3  OutDataTypeStr=fixdt(1,3,0)  SampleTime=-1
  Multiport Switch : MultiPortSwitch  DataPortOrder=Zero-based contiguous  Inputs=4  zeroidx=on
  I : Outport
  wires:
  Bit Slice2/1 -> Multiport Switch/1
  bits/1 -> Bit Slice2/1
  Constant3/1 -> Multiport Switch/3
  Constant4/1 -> Multiport Switch/2
  Constant1/1 -> Multiport Switch/4
  Constant2/1 -> Multiport Switch/5
  Multiport Switch/1 -> I/1

== system lib_rfsoc_fec/QAM Mapping/QAM Mapping/N-Width QAM-16 Symbol Mapping Real/QAM-16 Symbol Mapping 11 ==
  bits : Inport
  Bit Slice2 : hdlsllib/Logic and Bit Operations/Bit Slice  lidx=n+3  ridx=n+2
      settings: SourceProductBaseCode=SL
  Constant1 : Constant  Value=3  OutDataTypeStr=fixdt(1,3,0)  SampleTime=-1
  Constant2 : Constant  OutDataTypeStr=fixdt(1,3,0)  SampleTime=-1
  Constant3 : Constant  Value=-1  OutDataTypeStr=fixdt(1,3,0)  SampleTime=-1
  Constant4 : Constant  Value=-3  OutDataTypeStr=fixdt(1,3,0)  SampleTime=-1
  Multiport Switch : MultiPortSwitch  DataPortOrder=Zero-based contiguous  Inputs=4  zeroidx=on
  I : Outport
  wires:
  Bit Slice2/1 -> Multiport Switch/1
  bits/1 -> Bit Slice2/1
  Constant3/1 -> Multiport Switch/3
  Constant4/1 -> Multiport Switch/2
  Constant1/1 -> Multiport Switch/4
  Constant2/1 -> Multiport Switch/5
  Multiport Switch/1 -> I/1

== system lib_rfsoc_fec/QAM Mapping/QAM Mapping/N-Width QAM-16 Symbol Mapping Real/QAM-16 Symbol Mapping 12 ==
  bits : Inport
  Bit Slice2 : hdlsllib/Logic and Bit Operations/Bit Slice  lidx=n+3  ridx=n+2
      settings: SourceProductBaseCode=SL
  Constant1 : Constant  Value=3  OutDataTypeStr=fixdt(1,3,0)  SampleTime=-1
  Constant2 : Constant  OutDataTypeStr=fixdt(1,3,0)  SampleTime=-1
  Constant3 : Constant  Value=-1  OutDataTypeStr=fixdt(1,3,0)  SampleTime=-1
  Constant4 : Constant  Value=-3  OutDataTypeStr=fixdt(1,3,0)  SampleTime=-1
  Multiport Switch : MultiPortSwitch  DataPortOrder=Zero-based contiguous  Inputs=4  zeroidx=on
  I : Outport
  wires:
  Bit Slice2/1 -> Multiport Switch/1
  bits/1 -> Bit Slice2/1
  Constant3/1 -> Multiport Switch/3
  Constant4/1 -> Multiport Switch/2
  Constant1/1 -> Multiport Switch/4
  Constant2/1 -> Multiport Switch/5
  Multiport Switch/1 -> I/1

== system lib_rfsoc_fec/QAM Mapping/QAM Mapping/N-Width QAM-16 Symbol Mapping Real/QAM-16 Symbol Mapping 13 ==
  bits : Inport
  Bit Slice2 : hdlsllib/Logic and Bit Operations/Bit Slice  lidx=n+3  ridx=n+2
      settings: SourceProductBaseCode=SL
  Constant1 : Constant  Value=3  OutDataTypeStr=fixdt(1,3,0)  SampleTime=-1
  Constant2 : Constant  OutDataTypeStr=fixdt(1,3,0)  SampleTime=-1
  Constant3 : Constant  Value=-1  OutDataTypeStr=fixdt(1,3,0)  SampleTime=-1
  Constant4 : Constant  Value=-3  OutDataTypeStr=fixdt(1,3,0)  SampleTime=-1
  Multiport Switch : MultiPortSwitch  DataPortOrder=Zero-based contiguous  Inputs=4  zeroidx=on
  I : Outport
  wires:
  Bit Slice2/1 -> Multiport Switch/1
  bits/1 -> Bit Slice2/1
  Constant3/1 -> Multiport Switch/3
  Constant4/1 -> Multiport Switch/2
  Constant1/1 -> Multiport Switch/4
  Constant2/1 -> Multiport Switch/5
  Multiport Switch/1 -> I/1

== system lib_rfsoc_fec/QAM Mapping/QAM Mapping/N-Width QAM-16 Symbol Mapping Real/QAM-16 Symbol Mapping 14 ==
  bits : Inport
  Bit Slice2 : hdlsllib/Logic and Bit Operations/Bit Slice  lidx=n+3  ridx=n+2
      settings: SourceProductBaseCode=SL
  Constant1 : Constant  Value=3  OutDataTypeStr=fixdt(1,3,0)  SampleTime=-1
  Constant2 : Constant  OutDataTypeStr=fixdt(1,3,0)  SampleTime=-1
  Constant3 : Constant  Value=-1  OutDataTypeStr=fixdt(1,3,0)  SampleTime=-1
  Constant4 : Constant  Value=-3  OutDataTypeStr=fixdt(1,3,0)  SampleTime=-1
  Multiport Switch : MultiPortSwitch  DataPortOrder=Zero-based contiguous  Inputs=4  zeroidx=on
  I : Outport
  wires:
  Bit Slice2/1 -> Multiport Switch/1
  bits/1 -> Bit Slice2/1
  Constant3/1 -> Multiport Switch/3
  Constant4/1 -> Multiport Switch/2
  Constant1/1 -> Multiport Switch/4
  Constant2/1 -> Multiport Switch/5
  Multiport Switch/1 -> I/1

== system lib_rfsoc_fec/QAM Mapping/QAM Mapping/N-Width QAM-16 Symbol Mapping Real/QAM-16 Symbol Mapping 15 ==
  bits : Inport
  Bit Slice2 : hdlsllib/Logic and Bit Operations/Bit Slice  lidx=n+3  ridx=n+2
      settings: SourceProductBaseCode=SL
  Constant1 : Constant  Value=3  OutDataTypeStr=fixdt(1,3,0)  SampleTime=-1
  Constant2 : Constant  OutDataTypeStr=fixdt(1,3,0)  SampleTime=-1
  Constant3 : Constant  Value=-1  OutDataTypeStr=fixdt(1,3,0)  SampleTime=-1
  Constant4 : Constant  Value=-3  OutDataTypeStr=fixdt(1,3,0)  SampleTime=-1
  Multiport Switch : MultiPortSwitch  DataPortOrder=Zero-based contiguous  Inputs=4  zeroidx=on
  I : Outport
  wires:
  Bit Slice2/1 -> Multiport Switch/1
  bits/1 -> Bit Slice2/1
  Constant3/1 -> Multiport Switch/3
  Constant4/1 -> Multiport Switch/2
  Constant1/1 -> Multiport Switch/4
  Constant2/1 -> Multiport Switch/5
  Multiport Switch/1 -> I/1

== system lib_rfsoc_fec/QAM Mapping/QAM Mapping/N-Width QAM-16 Symbol Mapping Real/QAM-16 Symbol Mapping 16 ==
  bits : Inport
  Bit Slice2 : hdlsllib/Logic and Bit Operations/Bit Slice  lidx=n+3  ridx=n+2
      settings: SourceProductBaseCode=SL
  Constant1 : Constant  Value=3  OutDataTypeStr=fixdt(1,3,0)  SampleTime=-1
  Constant2 : Constant  OutDataTypeStr=fixdt(1,3,0)  SampleTime=-1
  Constant3 : Constant  Value=-1  OutDataTypeStr=fixdt(1,3,0)  SampleTime=-1
  Constant4 : Constant  Value=-3  OutDataTypeStr=fixdt(1,3,0)  SampleTime=-1
  Multiport Switch : MultiPortSwitch  DataPortOrder=Zero-based contiguous  Inputs=4  zeroidx=on
  I : Outport
  wires:
  Bit Slice2/1 -> Multiport Switch/1
  bits/1 -> Bit Slice2/1
  Constant3/1 -> Multiport Switch/3
  Constant4/1 -> Multiport Switch/2
  Constant1/1 -> Multiport Switch/4
  Constant2/1 -> Multiport Switch/5
  Multiport Switch/1 -> I/1

== system lib_rfsoc_fec/QAM Mapping/QAM Mapping/N-Width QAM-16 Symbol Mapping Real/QAM-16 Symbol Mapping 17 ==
  bits : Inport
  Bit Slice2 : hdlsllib/Logic and Bit Operations/Bit Slice  lidx=n+3  ridx=n+2
      settings: SourceProductBaseCode=SL
  Constant1 : Constant  Value=3  OutDataTypeStr=fixdt(1,3,0)  SampleTime=-1
  Constant2 : Constant  OutDataTypeStr=fixdt(1,3,0)  SampleTime=-1
  Constant3 : Constant  Value=-1  OutDataTypeStr=fixdt(1,3,0)  SampleTime=-1
  Constant4 : Constant  Value=-3  OutDataTypeStr=fixdt(1,3,0)  SampleTime=-1
  Multiport Switch : MultiPortSwitch  DataPortOrder=Zero-based contiguous  Inputs=4  zeroidx=on
  I : Outport
  wires:
  Bit Slice2/1 -> Multiport Switch/1
  bits/1 -> Bit Slice2/1
  Constant3/1 -> Multiport Switch/3
  Constant4/1 -> Multiport Switch/2
  Constant1/1 -> Multiport Switch/4
  Constant2/1 -> Multiport Switch/5
  Multiport Switch/1 -> I/1

== system lib_rfsoc_fec/QAM Mapping/QAM Mapping/N-Width QAM-16 Symbol Mapping Real/QAM-16 Symbol Mapping 18 ==
  bits : Inport
  Bit Slice2 : hdlsllib/Logic and Bit Operations/Bit Slice  lidx=n+3  ridx=n+2
      settings: SourceProductBaseCode=SL
  Constant1 : Constant  Value=3  OutDataTypeStr=fixdt(1,3,0)  SampleTime=-1
  Constant2 : Constant  OutDataTypeStr=fixdt(1,3,0)  SampleTime=-1
  Constant3 : Constant  Value=-1  OutDataTypeStr=fixdt(1,3,0)  SampleTime=-1
  Constant4 : Constant  Value=-3  OutDataTypeStr=fixdt(1,3,0)  SampleTime=-1
  Multiport Switch : MultiPortSwitch  DataPortOrder=Zero-based contiguous  Inputs=4  zeroidx=on
  I : Outport
  wires:
  Bit Slice2/1 -> Multiport Switch/1
  bits/1 -> Bit Slice2/1
  Constant3/1 -> Multiport Switch/3
  Constant4/1 -> Multiport Switch/2
  Constant1/1 -> Multiport Switch/4
  Constant2/1 -> Multiport Switch/5
  Multiport Switch/1 -> I/1

== system lib_rfsoc_fec/QAM Mapping/QAM Mapping/N-Width QAM-16 Symbol Mapping Real/QAM-16 Symbol Mapping 19 ==
  bits : Inport
  Bit Slice2 : hdlsllib/Logic and Bit Operations/Bit Slice  lidx=n+3  ridx=n+2
      settings: SourceProductBaseCode=SL
  Constant1 : Constant  Value=3  OutDataTypeStr=fixdt(1,3,0)  SampleTime=-1
  Constant2 : Constant  OutDataTypeStr=fixdt(1,3,0)  SampleTime=-1
  Constant3 : Constant  Value=-1  OutDataTypeStr=fixdt(1,3,0)  SampleTime=-1
  Constant4 : Constant  Value=-3  OutDataTypeStr=fixdt(1,3,0)  SampleTime=-1
  Multiport Switch : MultiPortSwitch  DataPortOrder=Zero-based contiguous  Inputs=4  zeroidx=on
  I : Outport
  wires:
  Bit Slice2/1 -> Multiport Switch/1
  bits/1 -> Bit Slice2/1
  Constant3/1 -> Multiport Switch/3
  Constant4/1 -> Multiport Switch/2
  Constant1/1 -> Multiport Switch/4
  Constant2/1 -> Multiport Switch/5
  Multiport Switch/1 -> I/1

== system lib_rfsoc_fec/QAM Mapping/QAM Mapping/N-Width QAM-16 Symbol Mapping Real/QAM-16 Symbol Mapping 2 ==
  bits : Inport
  Bit Slice2 : hdlsllib/Logic and Bit Operations/Bit Slice  lidx=n+3  ridx=n+2
      settings: SourceProductBaseCode=SL
  Constant1 : Constant  Value=3  OutDataTypeStr=fixdt(1,3,0)  SampleTime=-1
  Constant2 : Constant  OutDataTypeStr=fixdt(1,3,0)  SampleTime=-1
  Constant3 : Constant  Value=-1  OutDataTypeStr=fixdt(1,3,0)  SampleTime=-1
  Constant4 : Constant  Value=-3  OutDataTypeStr=fixdt(1,3,0)  SampleTime=-1
  Multiport Switch : MultiPortSwitch  DataPortOrder=Zero-based contiguous  Inputs=4  zeroidx=on
  I : Outport
  wires:
  Bit Slice2/1 -> Multiport Switch/1
  bits/1 -> Bit Slice2/1
  Constant3/1 -> Multiport Switch/3
  Constant4/1 -> Multiport Switch/2
  Constant1/1 -> Multiport Switch/4
  Constant2/1 -> Multiport Switch/5
  Multiport Switch/1 -> I/1

== system lib_rfsoc_fec/QAM Mapping/QAM Mapping/N-Width QAM-16 Symbol Mapping Real/QAM-16 Symbol Mapping 20 ==
  bits : Inport
  Bit Slice2 : hdlsllib/Logic and Bit Operations/Bit Slice  lidx=n+3  ridx=n+2
      settings: SourceProductBaseCode=SL
  Constant1 : Constant  Value=3  OutDataTypeStr=fixdt(1,3,0)  SampleTime=-1
  Constant2 : Constant  OutDataTypeStr=fixdt(1,3,0)  SampleTime=-1
  Constant3 : Constant  Value=-1  OutDataTypeStr=fixdt(1,3,0)  SampleTime=-1
  Constant4 : Constant  Value=-3  OutDataTypeStr=fixdt(1,3,0)  SampleTime=-1
  Multiport Switch : MultiPortSwitch  DataPortOrder=Zero-based contiguous  Inputs=4  zeroidx=on
  I : Outport
  wires:
  Bit Slice2/1 -> Multiport Switch/1
  bits/1 -> Bit Slice2/1
  Constant3/1 -> Multiport Switch/3
  Constant4/1 -> Multiport Switch/2
  Constant1/1 -> Multiport Switch/4
  Constant2/1 -> Multiport Switch/5
  Multiport Switch/1 -> I/1

== system lib_rfsoc_fec/QAM Mapping/QAM Mapping/N-Width QAM-16 Symbol Mapping Real/QAM-16 Symbol Mapping 21 ==
  bits : Inport
  Bit Slice2 : hdlsllib/Logic and Bit Operations/Bit Slice  lidx=n+3  ridx=n+2
      settings: SourceProductBaseCode=SL
  Constant1 : Constant  Value=3  OutDataTypeStr=fixdt(1,3,0)  SampleTime=-1
  Constant2 : Constant  OutDataTypeStr=fixdt(1,3,0)  SampleTime=-1
  Constant3 : Constant  Value=-1  OutDataTypeStr=fixdt(1,3,0)  SampleTime=-1
  Constant4 : Constant  Value=-3  OutDataTypeStr=fixdt(1,3,0)  SampleTime=-1
  Multiport Switch : MultiPortSwitch  DataPortOrder=Zero-based contiguous  Inputs=4  zeroidx=on
  I : Outport
  wires:
  Bit Slice2/1 -> Multiport Switch/1
  bits/1 -> Bit Slice2/1
  Constant3/1 -> Multiport Switch/3
  Constant4/1 -> Multiport Switch/2
  Constant1/1 -> Multiport Switch/4
  Constant2/1 -> Multiport Switch/5
  Multiport Switch/1 -> I/1

== system lib_rfsoc_fec/QAM Mapping/QAM Mapping/N-Width QAM-16 Symbol Mapping Real/QAM-16 Symbol Mapping 22 ==
  bits : Inport
  Bit Slice2 : hdlsllib/Logic and Bit Operations/Bit Slice  lidx=n+3  ridx=n+2
      settings: SourceProductBaseCode=SL
  Constant1 : Constant  Value=3  OutDataTypeStr=fixdt(1,3,0)  SampleTime=-1
  Constant2 : Constant  OutDataTypeStr=fixdt(1,3,0)  SampleTime=-1
  Constant3 : Constant  Value=-1  OutDataTypeStr=fixdt(1,3,0)  SampleTime=-1
  Constant4 : Constant  Value=-3  OutDataTypeStr=fixdt(1,3,0)  SampleTime=-1
  Multiport Switch : MultiPortSwitch  DataPortOrder=Zero-based contiguous  Inputs=4  zeroidx=on
  I : Outport
  wires:
  Bit Slice2/1 -> Multiport Switch/1
  bits/1 -> Bit Slice2/1
  Constant3/1 -> Multiport Switch/3
  Constant4/1 -> Multiport Switch/2
  Constant1/1 -> Multiport Switch/4
  Constant2/1 -> Multiport Switch/5
  Multiport Switch/1 -> I/1

== system lib_rfsoc_fec/QAM Mapping/QAM Mapping/N-Width QAM-16 Symbol Mapping Real/QAM-16 Symbol Mapping 23 ==
  bits : Inport
  Bit Slice2 : hdlsllib/Logic and Bit Operations/Bit Slice  lidx=n+3  ridx=n+2
      settings: SourceProductBaseCode=SL
  Constant1 : Constant  Value=3  OutDataTypeStr=fixdt(1,3,0)  SampleTime=-1
  Constant2 : Constant  OutDataTypeStr=fixdt(1,3,0)  SampleTime=-1
  Constant3 : Constant  Value=-1  OutDataTypeStr=fixdt(1,3,0)  SampleTime=-1
  Constant4 : Constant  Value=-3  OutDataTypeStr=fixdt(1,3,0)  SampleTime=-1
  Multiport Switch : MultiPortSwitch  DataPortOrder=Zero-based contiguous  Inputs=4  zeroidx=on
  I : Outport
  wires:
  Bit Slice2/1 -> Multiport Switch/1
  bits/1 -> Bit Slice2/1
  Constant3/1 -> Multiport Switch/3
  Constant4/1 -> Multiport Switch/2
  Constant1/1 -> Multiport Switch/4
  Constant2/1 -> Multiport Switch/5
  Multiport Switch/1 -> I/1

== system lib_rfsoc_fec/QAM Mapping/QAM Mapping/N-Width QAM-16 Symbol Mapping Real/QAM-16 Symbol Mapping 24 ==
  bits : Inport
  Bit Slice2 : hdlsllib/Logic and Bit Operations/Bit Slice  lidx=n+3  ridx=n+2
      settings: SourceProductBaseCode=SL
  Constant1 : Constant  Value=3  OutDataTypeStr=fixdt(1,3,0)  SampleTime=-1
  Constant2 : Constant  OutDataTypeStr=fixdt(1,3,0)  SampleTime=-1
  Constant3 : Constant  Value=-1  OutDataTypeStr=fixdt(1,3,0)  SampleTime=-1
  Constant4 : Constant  Value=-3  OutDataTypeStr=fixdt(1,3,0)  SampleTime=-1
  Multiport Switch : MultiPortSwitch  DataPortOrder=Zero-based contiguous  Inputs=4  zeroidx=on
  I : Outport
  wires:
  Bit Slice2/1 -> Multiport Switch/1
  bits/1 -> Bit Slice2/1
  Constant3/1 -> Multiport Switch/3
  Constant4/1 -> Multiport Switch/2
  Constant1/1 -> Multiport Switch/4
  Constant2/1 -> Multiport Switch/5
  Multiport Switch/1 -> I/1

== system lib_rfsoc_fec/QAM Mapping/QAM Mapping/N-Width QAM-16 Symbol Mapping Real/QAM-16 Symbol Mapping 25 ==
  bits : Inport
  Bit Slice2 : hdlsllib/Logic and Bit Operations/Bit Slice  lidx=n+3  ridx=n+2
      settings: SourceProductBaseCode=SL
  Constant1 : Constant  Value=3  OutDataTypeStr=fixdt(1,3,0)  SampleTime=-1
  Constant2 : Constant  OutDataTypeStr=fixdt(1,3,0)  SampleTime=-1
  Constant3 : Constant  Value=-1  OutDataTypeStr=fixdt(1,3,0)  SampleTime=-1
  Constant4 : Constant  Value=-3  OutDataTypeStr=fixdt(1,3,0)  SampleTime=-1
  Multiport Switch : MultiPortSwitch  DataPortOrder=Zero-based contiguous  Inputs=4  zeroidx=on
  I : Outport
  wires:
  Bit Slice2/1 -> Multiport Switch/1
  bits/1 -> Bit Slice2/1
  Constant3/1 -> Multiport Switch/3
  Constant4/1 -> Multiport Switch/2
  Constant1/1 -> Multiport Switch/4
  Constant2/1 -> Multiport Switch/5
  Multiport Switch/1 -> I/1

== system lib_rfsoc_fec/QAM Mapping/QAM Mapping/N-Width QAM-16 Symbol Mapping Real/QAM-16 Symbol Mapping 26 ==
  bits : Inport
  Bit Slice2 : hdlsllib/Logic and Bit Operations/Bit Slice  lidx=n+3  ridx=n+2
      settings: SourceProductBaseCode=SL
  Constant1 : Constant  Value=3  OutDataTypeStr=fixdt(1,3,0)  SampleTime=-1
  Constant2 : Constant  OutDataTypeStr=fixdt(1,3,0)  SampleTime=-1
  Constant3 : Constant  Value=-1  OutDataTypeStr=fixdt(1,3,0)  SampleTime=-1
  Constant4 : Constant  Value=-3  OutDataTypeStr=fixdt(1,3,0)  SampleTime=-1
  Multiport Switch : MultiPortSwitch  DataPortOrder=Zero-based contiguous  Inputs=4  zeroidx=on
  I : Outport
  wires:
  Bit Slice2/1 -> Multiport Switch/1
  bits/1 -> Bit Slice2/1
  Constant3/1 -> Multiport Switch/3
  Constant4/1 -> Multiport Switch/2
  Constant1/1 -> Multiport Switch/4
  Constant2/1 -> Multiport Switch/5
  Multiport Switch/1 -> I/1

== system lib_rfsoc_fec/QAM Mapping/QAM Mapping/N-Width QAM-16 Symbol Mapping Real/QAM-16 Symbol Mapping 27 ==
  bits : Inport
  Bit Slice2 : hdlsllib/Logic and Bit Operations/Bit Slice  lidx=n+3  ridx=n+2
      settings: SourceProductBaseCode=SL
  Constant1 : Constant  Value=3  OutDataTypeStr=fixdt(1,3,0)  SampleTime=-1
  Constant2 : Constant  OutDataTypeStr=fixdt(1,3,0)  SampleTime=-1
  Constant3 : Constant  Value=-1  OutDataTypeStr=fixdt(1,3,0)  SampleTime=-1
  Constant4 : Constant  Value=-3  OutDataTypeStr=fixdt(1,3,0)  SampleTime=-1
  Multiport Switch : MultiPortSwitch  DataPortOrder=Zero-based contiguous  Inputs=4  zeroidx=on
  I : Outport
  wires:
  Bit Slice2/1 -> Multiport Switch/1
  bits/1 -> Bit Slice2/1
  Constant3/1 -> Multiport Switch/3
  Constant4/1 -> Multiport Switch/2
  Constant1/1 -> Multiport Switch/4
  Constant2/1 -> Multiport Switch/5
  Multiport Switch/1 -> I/1

== system lib_rfsoc_fec/QAM Mapping/QAM Mapping/N-Width QAM-16 Symbol Mapping Real/QAM-16 Symbol Mapping 28 ==
  bits : Inport
  Bit Slice2 : hdlsllib/Logic and Bit Operations/Bit Slice  lidx=n+3  ridx=n+2
      settings: SourceProductBaseCode=SL
  Constant1 : Constant  Value=3  OutDataTypeStr=fixdt(1,3,0)  SampleTime=-1
  Constant2 : Constant  OutDataTypeStr=fixdt(1,3,0)  SampleTime=-1
  Constant3 : Constant  Value=-1  OutDataTypeStr=fixdt(1,3,0)  SampleTime=-1
  Constant4 : Constant  Value=-3  OutDataTypeStr=fixdt(1,3,0)  SampleTime=-1
  Multiport Switch : MultiPortSwitch  DataPortOrder=Zero-based contiguous  Inputs=4  zeroidx=on
  I : Outport
  wires:
  Bit Slice2/1 -> Multiport Switch/1
  bits/1 -> Bit Slice2/1
  Constant3/1 -> Multiport Switch/3
  Constant4/1 -> Multiport Switch/2
  Constant1/1 -> Multiport Switch/4
  Constant2/1 -> Multiport Switch/5
  Multiport Switch/1 -> I/1

== system lib_rfsoc_fec/QAM Mapping/QAM Mapping/N-Width QAM-16 Symbol Mapping Real/QAM-16 Symbol Mapping 29 ==
  bits : Inport
  Bit Slice2 : hdlsllib/Logic and Bit Operations/Bit Slice  lidx=n+3  ridx=n+2
      settings: SourceProductBaseCode=SL
  Constant1 : Constant  Value=3  OutDataTypeStr=fixdt(1,3,0)  SampleTime=-1
  Constant2 : Constant  OutDataTypeStr=fixdt(1,3,0)  SampleTime=-1
  Constant3 : Constant  Value=-1  OutDataTypeStr=fixdt(1,3,0)  SampleTime=-1
  Constant4 : Constant  Value=-3  OutDataTypeStr=fixdt(1,3,0)  SampleTime=-1
  Multiport Switch : MultiPortSwitch  DataPortOrder=Zero-based contiguous  Inputs=4  zeroidx=on
  I : Outport
  wires:
  Bit Slice2/1 -> Multiport Switch/1
  bits/1 -> Bit Slice2/1
  Constant3/1 -> Multiport Switch/3
  Constant4/1 -> Multiport Switch/2
  Constant1/1 -> Multiport Switch/4
  Constant2/1 -> Multiport Switch/5
  Multiport Switch/1 -> I/1

== system lib_rfsoc_fec/QAM Mapping/QAM Mapping/N-Width QAM-16 Symbol Mapping Real/QAM-16 Symbol Mapping 3 ==
  bits : Inport
  Bit Slice2 : hdlsllib/Logic and Bit Operations/Bit Slice  lidx=n+3  ridx=n+2
      settings: SourceProductBaseCode=SL
  Constant1 : Constant  Value=3  OutDataTypeStr=fixdt(1,3,0)  SampleTime=-1
  Constant2 : Constant  OutDataTypeStr=fixdt(1,3,0)  SampleTime=-1
  Constant3 : Constant  Value=-1  OutDataTypeStr=fixdt(1,3,0)  SampleTime=-1
  Constant4 : Constant  Value=-3  OutDataTypeStr=fixdt(1,3,0)  SampleTime=-1
  Multiport Switch : MultiPortSwitch  DataPortOrder=Zero-based contiguous  Inputs=4  zeroidx=on
  I : Outport
  wires:
  Bit Slice2/1 -> Multiport Switch/1
  bits/1 -> Bit Slice2/1
  Constant3/1 -> Multiport Switch/3
  Constant4/1 -> Multiport Switch/2
  Constant1/1 -> Multiport Switch/4
  Constant2/1 -> Multiport Switch/5
  Multiport Switch/1 -> I/1

== system lib_rfsoc_fec/QAM Mapping/QAM Mapping/N-Width QAM-16 Symbol Mapping Real/QAM-16 Symbol Mapping 30 ==
  bits : Inport
  Bit Slice2 : hdlsllib/Logic and Bit Operations/Bit Slice  lidx=n+3  ridx=n+2
      settings: SourceProductBaseCode=SL
  Constant1 : Constant  Value=3  OutDataTypeStr=fixdt(1,3,0)  SampleTime=-1
  Constant2 : Constant  OutDataTypeStr=fixdt(1,3,0)  SampleTime=-1
  Constant3 : Constant  Value=-1  OutDataTypeStr=fixdt(1,3,0)  SampleTime=-1
  Constant4 : Constant  Value=-3  OutDataTypeStr=fixdt(1,3,0)  SampleTime=-1
  Multiport Switch : MultiPortSwitch  DataPortOrder=Zero-based contiguous  Inputs=4  zeroidx=on
  I : Outport
  wires:
  Bit Slice2/1 -> Multiport Switch/1
  bits/1 -> Bit Slice2/1
  Constant3/1 -> Multiport Switch/3
  Constant4/1 -> Multiport Switch/2
  Constant1/1 -> Multiport Switch/4
  Constant2/1 -> Multiport Switch/5
  Multiport Switch/1 -> I/1

== system lib_rfsoc_fec/QAM Mapping/QAM Mapping/N-Width QAM-16 Symbol Mapping Real/QAM-16 Symbol Mapping 31 ==
  bits : Inport
  Bit Slice2 : hdlsllib/Logic and Bit Operations/Bit Slice  lidx=n+3  ridx=n+2
      settings: SourceProductBaseCode=SL
  Constant1 : Constant  Value=3  OutDataTypeStr=fixdt(1,3,0)  SampleTime=-1
  Constant2 : Constant  OutDataTypeStr=fixdt(1,3,0)  SampleTime=-1
  Constant3 : Constant  Value=-1  OutDataTypeStr=fixdt(1,3,0)  SampleTime=-1
  Constant4 : Constant  Value=-3  OutDataTypeStr=fixdt(1,3,0)  SampleTime=-1
  Multiport Switch : MultiPortSwitch  DataPortOrder=Zero-based contiguous  Inputs=4  zeroidx=on
  I : Outport
  wires:
  Bit Slice2/1 -> Multiport Switch/1
  bits/1 -> Bit Slice2/1
  Constant3/1 -> Multiport Switch/3
  Constant4/1 -> Multiport Switch/2
  Constant1/1 -> Multiport Switch/4
  Constant2/1 -> Multiport Switch/5
  Multiport Switch/1 -> I/1
